simulink subsystem "FTC_UnknownV4"  (R2022a)
settings: Solver=VariableStepAuto  StartTime=0.0  StopTime=10.0  RelTol=1e-3
values from neighbouring files (symbols this model uses):
  g = (9.8)    (= 9.8)    [H250_LOEKnown_400HzParam.m]    (also in H250_LOEUnknown_400HzParam.m; H333_LOEKnown_400HzParam.m)
  J = (diag([0.0056 0.0056 0.0104]))    [H250_LOEKnown_400HzParam.m]    (also in H250_LOEUnknown_400HzParam.m; H333_LOEKnown_400HzParam.m = (diag([0.012 0.0120 0.02])))
  M = ([ 1          1          1         1 ... (first row only)    [H250_LOEKnown_400HzParam.m]    (also in H250_LOEUnknown_400HzParam.m; H333_LOEKnown_400HzParam.m)
  m = (0.752)    (= 0.752)    [H250_LOEKnown_400HzParam.m]    (also in H250_LOEUnknown_400HzParam.m; H333_LOEKnown_400HzParam.m = 1.13)
  MY_ATT_P = Pixhawk_CSC.Parameter( {single(8), 'MY_ATT_P'}  )    [H250_LOEKnown_400HzParam.m]    (also in H250_LOEUnknown_400HzParam.m = Pixhawk_CSC.Parameter( {single(3), 'MY_ATT_P'}  ); H333_LOEKnown_400HzParam.m)
  MY_ATT_P_YAW = Pixhawk_CSC.Parameter( {single(0), 'MY_ATT_P_YAW'}  )    [H250_LOEKnown_400HzParam.m]    (also in H250_LOEUnknown_400HzParam.m = Pixhawk_CSC.Parameter( {single(0.0), 'MY_ATT_P_YAW'}  ); H333_LOEKnown_400HzParam.m)
  MY_K_CP = Pixhawk_CSC.Parameter({single(0.7), 'MY_K_CP'} )    [H250_LOEUnknown_400HzParam.m]
  MY_POS_P = Pixhawk_CSC.Parameter( {single(0.5), 'MY_POS_P'}  )    [H250_LOEKnown_400HzParam.m]    (also in H250_LOEUnknown_400HzParam.m; H333_LOEKnown_400HzParam.m)
  MY_RATE_P = Pixhawk_CSC.Parameter( {single(12), 'MY_RATE_P'}  )    [H250_LOEKnown_400HzParam.m]    (also in H250_LOEUnknown_400HzParam.m = Pixhawk_CSC.Parameter( {single(14), 'MY_RATE_P'}  ); H333_LOEKnown_400HzParam.m)
  MY_RATE_P_YAW = Pixhawk_CSC.Parameter( {single(0.3), 'MY_RATE_P_YAW'}  )    [H250_LOEKnown_400HzParam.m]    (also in H250_LOEUnknown_400HzParam.m = Pixhawk_CSC.Parameter( {single(0.0), 'MY_RATE_P_YAW'}  ); H333_LOEKnown_400HzParam.m)
  MY_SAT_AD = Pixhawk_CSC.Parameter({single(0.13), 'MY_SAT_AD'} )    [H250_LOEKnown_400HzParam.m]    (also in H250_LOEUnknown_400HzParam.m; H333_LOEKnown_400HzParam.m)
  MY_TAU_P_A = Pixhawk_CSC.Parameter( {single(0), 'MY_TAU_P_A'}  )    [H250_LOEKnown_400HzParam.m]    (also in H250_LOEUnknown_400HzParam.m = Pixhawk_CSC.Parameter( {single(0.0), 'MY_TAU_P_A'}  ); H333_LOEKnown_400HzParam.m)
  MY_TAU_P_A_YAW = Pixhawk_CSC.Parameter( {single(0), 'MY_TAU_P_A_YAW'}  )    [H250_LOEKnown_400HzParam.m]    (also in H250_LOEUnknown_400HzParam.m; H333_LOEKnown_400HzParam.m)
  MY_TAU_P_P = Pixhawk_CSC.Parameter( {single(1.5), 'MY_TAU_P_P'}  )    [H250_LOEKnown_400HzParam.m]    (also in H250_LOEUnknown_400HzParam.m = Pixhawk_CSC.Parameter( {single(1.3), 'MY_TAU_P_P'}  ); H333_LOEKnown_400HzParam.m)
  MY_TAU_P_P_YAW = Pixhawk_CSC.Parameter( {single(0.1), 'MY_TAU_P_P_YAW'}  )    [H250_LOEKnown_400HzParam.m]    (also in H250_LOEUnknown_400HzParam.m; H333_LOEKnown_400HzParam.m)
  MY_VEL_P = Pixhawk_CSC.Parameter( {single(0.8), 'MY_VEL_P'}  )    [H250_LOEKnown_400HzParam.m]    (also in H250_LOEUnknown_400HzParam.m; H333_LOEKnown_400HzParam.m)
  T00 = single([m*g/4 m*g/4 m*g/4 m*g/4]')    [H250_LOEKnown_400HzParam.m]    (also in H250_LOEUnknown_400HzParam.m; H333_LOEKnown_400HzParam.m)
  Tf = 0.06    [H250_LOEKnown_400HzParam.m]    (also in H250_LOEUnknown_400HzParam.m; H333_LOEKnown_400HzParam.m)
  Tmotorbar = (0.035)    (= 0.035)    [H250_LOEKnown_400HzParam.m]    (also in H250_LOEUnknown_400HzParam.m = 0.032; H333_LOEKnown_400HzParam.m)
  Ts = 1/400    (= 0.0025)    [H250_LOEKnown_400HzParam.m]    (also in H250_LOEUnknown_400HzParam.m; H333_LOEKnown_400HzParam.m)
undefined symbols (not defined in the file or in its folder): MY_POS_ALT, MY_VEL_ALT
libraries: discretizing x14, slpidlib x4, simulink x2, pixhawk_slib_uORB_RW x1
(part 2 of 2)

== matlab function FTC_UnknownV4/quat2eul1 ==
  data: q input single; dcm output single
function dcm  = quat2eul(q)
% Conversion from Quaternion to Euler angles based on the PX4 Firmware
% v1.6.5 release.
% 
% Quaternion -> DCM -> Euler Angles
% INPUT:
%   q: Quaternion vector of the format: (a + bi + cj + dk)
% OUTPUT:
%   [phi,theta,psi]: Euler angles in radians.
% 
 if norm(q)~=0
    a = q(1);
    b = q(2);
    c = q(3);
    d = q(4);

    aSq = a*a;
    bSq = b*b;
    cSq = c*c;
    dSq = d*d;

    d_pi2 = pi/2;

    % quaternion_to_dcm
    dcm00 = aSq + bSq - cSq - dSq;
    dcm01 = 2*(b*c - a*d);
    dcm02 = 2*(a*c + b*d);
    dcm10 = 2*(b*c + a*d);
    dcm11 = aSq - bSq + cSq - dSq;
    dcm12 = 2*(c*d - a*b);
    dcm20 = 2*(b*d - a*c);
    dcm21 = 2*(a*b + c*d);
    dcm22 = aSq - bSq - cSq + dSq;
    dcm=[dcm00 dcm01 dcm02;
              dcm10 dcm11 dcm12;
              dcm20 dcm21  dcm22];
 else
     dcm = single(eye(3,3));
 end
    % dcm_to_euler

== matlab function FTC_UnknownV4/innerloop/AttRate ==
  data: pqrd input; w input; dw input; T_ input; M input; RATE_P input; RATE_P_YAW input; J input; dpqr output size=3; taop output; taoq output; taor output; K_CP input
function [dpqr, taop, taoq, taor] = fcn(pqrd, w, dw, T_, M, RATE_P, RATE_P_YAW, J, K_CP)
pqd = pqrd(1:2);
rd    = pqrd(3);
%% 角速率控制器计算

k2 = RATE_P;
k2_scaled = k2*RATE_P_YAW;

% kr = 0.001;
% dp =  M(2,:)*T_ - J(1,1)*dw(1) - kr*abs(w(1))*w(1) + w(2)*w(3)*(J(2,2)-J(3,3));
% dq =  M(3,:)*T_ - J(2,2)*dw(2) - kr*abs(w(2))*w(2) + w(3)*w(1)*(J(3,3)-J(1,1));
% dr  =  M(4,:)*T_ - J(3,3)*dw(3) - kr*abs(w(3))*w(3) + w(1)*w(2)*(J(1,1)-J(2,2));
dp = M(2,:)*T_ -J(1,1)*dw(1) + w(2)*w(3)*(J(2,2)-J(3,3));
dq = M(3,:)*T_ -J(2,2)*dw(2) + w(3)*w(1)*(J(3,3)-J(1,1));
dr = M(4,:)*T_ -J(3,3)*dw(3);

% taop =            J(1,1)*k2*(pqd(1)-w(1)) + kr*abs(w(1))*w(1) - w(2)*w(3)*(J(2,2)-J(3,3))+dp;
% taoq =            J(2,2)*k2*(pqd(2)-w(2)) + kr*abs(w(2))*w(2) - w(3)*w(1)*(J(3,3)-J(1,1))+dq;
% taor  = mysatsingle(J(3,3)*k2_scaled*(rd-w(3)) + kr*abs(w(3))*w(3) - w(1)*w(2)*(J(1,1)-J(2,2))+dr,10.0);

% 叠加耦合项 -\omega\times J\omega
taop =           J(1,1)*k2*(pqd(1)-w(1)) - w(2)*w(3)*(J(2,2)-J(3,3)) + dp + K_CP*w(2)*w(3)*(J(2,2)-J(3,3));
taoq =           J(2,2)*k2*(pqd(2)-w(2)) - w(3)*w(1)*(J(3,3)-J(1,1)) + dq + K_CP*w(3)*w(1)*(J(3,3)-J(1,1));
taor  = mysatsingle(J(3,3)*k2_scaled*(rd-w(3))+ dr,1.0);

dpqr = [dp; dq; dr];

== matlab function FTC_UnknownV4/MATLAB Function4 ==
  data: x input; y2 output
function y2 = fcn(x)
p1 = 19.72;
p2 = -134.1;
p3 = 385.9;
y=p1*x.^2 + p2.*x + p3;
y2 = y.*x;

== matlab function FTC_UnknownV4/innerloop/fmincon ==
  data: fd input; taop input; taoq input; taor input; T output; T0 input; M input; val output; time output
function [T,val,time] = fcn(fd, taop, taoq, taor, T0, M)
%% 求解
w1= 1;
w2 =20;
w3= 20;
w4= 0.00;
myfun2 = @(x)(w1*(M(1,:)*x-fd)^2+w2*(M(2,:)*x-taop)^2+w3*(M(3,:)*x-taoq)^2+w4*(M(4,:)*x-taor)^2);

lb  = [0 0 0 0]';
ub  = [3 3 3 3]';

options = optimoptions(@fmincon,'Algorithm','sqp','MaxIterations',10);
% tic
[T,val] = fmincon(myfun2,T0,[],[],[],[],lb,ub,[],options);
% ff = toc;
time =0;

== matlab function FTC_UnknownV4/innerloop/quadprog ==
  data: fd input double; taop input double; taoq input double; taor input double; T output double; T0 input double; M input double; fval output double; iter output
function [T,fval, iter] = fcn(fd, taop, taoq, taor, T0, M)
%% 求解
vd = [fd; taop; taoq; taor];
W=diag([1 20 20 0.01]);
H = M'*W*M;
f = -(vd'*W*M)';
% Td = B*vd;
lb  = [0 0 0 0]';
ub  = [8.5 8.5 8.5 8.5]';
% if (max(B*vd)>3)||(min(B*vd)<0)
    options = optimoptions(@quadprog,'Algorithm','active-set','MaxIterations',10);

    [T,fval,~,output] = quadprog(H, f, [], [], [], [], lb, ub, T0, options);
     iter = output.iterations;
% else
%     T = B*vd;
%     fval = 0;
% end

== matlab function FTC_UnknownV4/innerloop/MATLAB Function1 ==
  data: u input; y output
function y = fcn(u)
y=diag([u,1,1,1]);

== matlab function FTC_UnknownV4/InputConditioning/MATLAB Function ==
  data: u input; y output
function y = fcn(u)

 if(u>1550)
    y=u;
 else
     if(u<1450)
     y=u;
     else
         y=single(1500);
     end
 end

== matlab function FTC_UnknownV4/InputConditioning/MATLAB Function1 ==
  data: u input; y output
function y = fcn(u)

 if(u>1550)
    y=u;
 else
     if(u<1450)
     y=u;
     else
         y=single(1500);
     end
 end

== matlab function FTC_UnknownV4/InputConditioning/MATLAB Function2 ==
  data: u input; y output
function y = fcn(u)

 if(u>1550)
    y=u;
 else
     if(u<1450)
     y=u;
     else
         y=single(1500);
     end
 end

== matlab function FTC_UnknownV4/MATLAB Function ==
  data: Lambda input; y output; fadePWM input
function y = fcn(Lambda, fadePWM)
s1 = Lambda(1,1) + Lambda(2,2) + Lambda(3,3) + Lambda(4,4);
if s1 ==1
    fadePWM(fadePWM==0)=170;
%     if(fadePWM(1)==0)
%         fadePWM(1) = 100;
%     end
%     if(fadePWM(1)==0)
%         fadePWM(1) = 100;
%     end
%     if(fadePWM(1)==0)
%         fadePWM(1) = 100;
%     end
%     if(fadePWM(4)==0)
%         fadePWM(4) = 100;
%     end
end
y = fadePWM+1000;

== matlab function FTC_UnknownV4/innerloop/Att ==
  data: e input; w input; eulerangle input; pqrd output; ATT_P input; ATT_P_SCALE input
function pqrd  = fcn(e, w, eulerangle, ATT_P, ATT_P_SCALE)
%% 角度控制1
% h1 = n3(1);
% h2 = n3(2);
% h3 = n3(3);
% h1d = n3d(1);
% h2d = n3d(2);
% h3d = n3d(3);
% we = Reb*w;
% k1 = single(5);
% epqd = [0 -1/h3; 1/h3 0]*[k1*(h1d-h1)+h2*we(3);k1*(h2d-h2)-h1*we(3)];
% 
% psid = single(0);
% rd = k1*0.3*(psid - psi);
% 
% Rbe = Reb';
% erd = (rd - Rbe(3,1)*epqd(1) - Rbe(3,2)*epqd(2))/Rbe(3,3);
% 
% pqd = Rbe((1:2),:)*[epqd; erd];%计算出机体系下的pqd
% pqd = mysat(pqd,2);
% pqrd = [pqd;rd];
%% 角度控制2
e1 = e(1);
e2 = e(2);
% e1  = n3(1) - n3d(1);
% e2  = n3(2) - n3d(2); 
beta = atan2(e2,e1);
psi = eulerangle(1);
costheta = eulerangle(2);
cosphi = eulerangle(3);
k1 = ATT_P;
pqd = [ -k1*sqrt(e1^2+e2^2)*sin(psi-beta);%costheta
             -k1*sqrt(e1^2+e2^2)*cos(psi-beta)];%cosphi
pqd = mysatsingle(pqd,3);
psid = 0;
% rd = -k1*0.3*(psi-psid);
rd = -k1*ATT_P_SCALE*(psi-psid);
% rd = 0;
pqrd = [pqd;rd];

== matlab function FTC_UnknownV4/innerloop/MATLAB Function2 ==
  data: pqd output; dpqr output; J input; Reb input; n3 input; n3d input; dn3d input; taop output; wf input; euler input; ATT_P_SCALE input; ATT_P input; f_dyn_m input; tilde_v input; dw input; T_ input; M input; K_CP input; RATE_P_YAW input; RATE_P input; taoq output; taor output
function [pqd,dpqr, taop, taoq, taor] = fcn(J, Reb, n3, n3d, dn3d, wf, euler, ATT_P_SCALE, ATT_P, f_dyn_m, tilde_v, dw, T_, M, K_CP, RATE_P_YAW, RATE_P)
A = Reb(1,1);
B = Reb(2,1);
C = Reb(1,2);
D = Reb(2,2);
E = Reb(3,1);
F = Reb(3,2);
n_3_x = Reb(1,3);
n_3_y = Reb(2,3);
n_3_z = Reb(3,3);
fx_1 = ([0 n_3_z;-n_3_z 0]*[A C;B D] + [-n_3_y;n_3_x]*[E F]);
K = ATT_P*[-B A;-D C];
G = -n_3_z*ATT_P*[1 0;0 1];
% For dotK
dReb = Reb*[0 -wf(3) wf(2);wf(3) 0 -wf(1);-wf(2) wf(1) 0];
dA = dReb(1,1);
dB = dReb(2,1);
dC = dReb(1,2);
dD = dReb(2,2);
dK = ATT_P*[-dB dA;-dD dC];
% For A_2
A_2 = [0 -wf(3)*(J(3,3)-J(2,2))/J(1,1);-wf(3)*(J(1,1)-J(3,3))/J(2,2) 0];

%% Controller
e = n3 - n3d;
% % Attitude Loop
%pqd = K*e(1:2);%期望主轴为常值的时候
pqd = K*e(1:2) + (K/ATT_P/(-n_3_z))*dn3d(1:2) + (K/ATT_P/(-n3(3)))*f_dyn_m*tilde_v;%考虑期望的主轴为动态变化的时候
rd = -ATT_P*ATT_P_SCALE*(euler(1));
% % Rate Loop generating u_c
u_cpq = [J(1,1) 0;0 J(2,2)]*(-RATE_P*(wf(1:2)-pqd)-A_2*wf(1:2)-(fx_1'-dK-G*K)*e(1:2) + G*(wf(1:2)-pqd));%-(fx_1'-dK-G*K)*e(1:2) + G*(wf(1:2)-pqd)
u_cr  = J(3,3)*RATE_P*RATE_P_YAW*(rd-wf(3));

% Disturbance Estimate d
dp = M(2,:)*T_ -J(1,1)*dw(1) + wf(2)*wf(3)*(J(2,2)-J(3,3));
dq = M(3,:)*T_ -J(2,2)*dw(2) + wf(3)*wf(1)*(J(3,3)-J(1,1));
dr  = M(4,:)*T_ -J(3,3)*dw(3);
dpqr = [dp; dq; dr];

% u_0 = u_c + d
taop = u_cpq(1) + dp + K_CP*(wf(2) - pqd(2))*wf(3)*(J(2,2)-J(3,3));
taoq = u_cpq(2) + dq + K_CP*(wf(1) - pqd(1))*wf(3)*(J(3,3)-J(1,1));
taor = mysatsingle(u_cr + dr,1.0);

== matlab function FTC_UnknownV4/outerloop/Position2/MATLAB Function ==
  data: manualRC input; pos_d output; current_pos input; Ts input
function pos_d = fcn(manualRC, current_pos, Ts)
persistent desired_pos_static manualRC_last
if isempty(desired_pos_static)
    desired_pos_static = current_pos;
end
if isempty(manualRC_last)
    manualRC_last = single([0;0]);
end

if norm(manualRC)>0.01
    desired_pos_static = desired_pos_static + Ts*manualRC;
else
    if manualRC_last>0.01
        desired_pos_static = current_pos;
    end
end
manualRC_last = manualRC;
pos_d = desired_pos_static;
